simulink model "test_com_SensorFusion_SF_D4_slip_GPS_ukf"  (R2019b)
settings: Solver=FixedStepDiscrete  StartTime=0  StopTime=stop  FixedStep=0.001  RelTol=1e-3
undefined symbols (not defined in the file or in its folder): BxTM, ByTM, CxTM, CyTM, g, gamma_stat_front, gamma_stat_rear, gearbox_ratio, l_F, l_R, m_sprung, m_unsprung_quarter, mag_calib_front_center, mag_calib_front_compmatrix, mag_calib_rear_center, mag_calib_rear_compmatrix, should_be_in_theSensorFusion, switch_VelYcalculation_pSF, testStart_VelX_pSF, testVelY_pSF, tire_r_dyn, track_angle_front, track_width_front, track_width_rear, v2o_x, wheel_kinematics_breakpoints, wheel_kinematics_FL_data, wheel_kinematics_FR_data, wheelbase, x9DFrontX, x9DFrontY, x9DRearX, x9DRearY
libraries: SignalProcessingSensorFusionLib x30, simulink x6
(part 6 of 8)

== matlab function test_com_SensorFusion_SF_D4_slip_GPS_ukf/Subsystem14/SensorFusion_E10/kalman ==
  data: YawRateCalculated output; x9DFront input; x9DRear input; VehicleState output Bus: control_VehicleState size=1; state output single size=22; Covariance output single; v2o input; WheelSpeeds input; WheelSpeeds_Sq input; RockerAngle input; RockerAngle_Sq input; dt input; x9DFrontX parameter; x9DRearX parameter; v2o_x parameter; track_width_front parameter; track_width_rear parameter; z_output output single; TireLoad output; m_sprung parameter; m_unsprung_quarter parameter; l_R parameter; l_F parameter; wheelbase parameter; h_cg parameter; motion_ratio_front parameter; motion_ratio_rear parameter; motion_ratio_heave_front parameter; motion_ratio_heave_rear parameter; motion_ratio_roll_front parameter; motion_ratio_roll_rear parameter; spring_stiff_heave_front parameter; spring_stiff_heave_rear parameter; spring_stiff_roll_front parameter; spring_stiff_roll_rear parameter; damp_coef_heave_front_push parameter size=[1 3]; damp_coef_heave_front_pull parameter size=[1 3]; damp_coef_heave_rear_push parameter size=[1 3]; damp_coef_heave_rear_pull parameter size=[1 3]; damp_coef_roll_front_push parameter size=[1 3]; damp_coef_roll_front_pull parameter size=[1 3]; damp_coef_roll_rear_push parameter size=[1 3]; damp_coef_roll_rear_pull parameter size=[1 3]; g parameter; tire_r_dyn parameter; delta input; Output output; TireSlipLong output; TireSlipAngle output; bias output; measurements_nb_out output; Position_out output; WheelAngle_FL input; WheelAngle_FR input; RockerAngle_nb output; WheelVelocity output; Fx_wheel_wheel input single size=4; Fy_wheel_wheel input single size=4; c_Reib input; rho_air parameter; cdA parameter; clA_front parameter; clA_rear parameter; x9D_Front_AccX_nb output; x9D_Rear_AccX_nb output; kalman_is_running output; switch_VelYcalculation_pSF input; testVelY_pSF input; testStart_VelX_pSF input
function [YawRateCalculated, VehicleState, state, Covariance, z_output , TireLoad, Output, TireSlipLong, TireSlipAngle,...
    bias,measurements_nb_out,Position_out, ...
    RockerAngle_nb, WheelVelocity, x9D_Front_AccX_nb, x9D_Rear_AccX_nb, kalman_is_running]    ...										
    = kalman(x9DFront, x9DRear, v2o, WheelSpeeds, WheelSpeeds_Sq, RockerAngle, RockerAngle_Sq,...
    dt, x9DFrontX, x9DRearX, v2o_x, track_width_front, track_width_rear, ...
    m_sprung,  m_unsprung_quarter, l_R, l_F, wheelbase, h_cg, motion_ratio_front, motion_ratio_rear, ...
    motion_ratio_heave_front, motion_ratio_heave_rear, motion_ratio_roll_front, motion_ratio_roll_rear, ...
    spring_stiff_heave_front, spring_stiff_heave_rear, spring_stiff_roll_front, spring_stiff_roll_rear, ...
    damp_coef_heave_front_push, damp_coef_heave_front_pull, damp_coef_heave_rear_push, damp_coef_heave_rear_pull,...
    damp_coef_roll_front_push, damp_coef_roll_front_pull, damp_coef_roll_rear_push, damp_coef_roll_rear_pull, ...
    g, tire_r_dyn, delta, WheelAngle_FL, WheelAngle_FR, Fx_wheel_wheel, Fy_wheel_wheel,...
    c_Reib, rho_air, cdA, clA_front, clA_rear, switch_VelYcalculation_pSF, testVelY_pSF, testStart_VelX_pSF)


persistent x P
%persistent x_TireLoad P_TireLoad
									
persistent WheelSpeedsCloseTogether_counter WheelSpeedsNoJump_counter
persistent WheelVelocity_old yawRate_old rollAng_old pitchAng_old PosZ_old v2o_VelX_old
persistent TireLoad_old

%Variablen für bias Messung
persistent standstill_counter
persistent bias_measurements 
persistent P_bias



%% Setup

% kalman filter
% x_k+1 = F x_k + w_k
% z_k = H x_k + v_k

% State vector 

% x = [ PosX;           % (1)   x-coordinate of the car  
%       VelX;           % (2)   Velocity of the car in x-direction 
%       AccX;           % (3)   Acceleration in x-direction of the car (CG) 
%       PosY;           % (4)   y-coordinate of the car 
%       VelY;           % (5)   Velocity of the car in y-direction 
%       AccY;           % (6)   Acceleration in y-direction of the car (CG) 
%       PosZ;           % (7)   z-coordinate of the car 
%       VelZ;           % (8)   Velocity of the car in z-direction 
%       AccZ;           % (9)   Acceleration in z-direction of the car (CG) 
%       RollAng;        % (10)  RollAngle of the Monocoque 
%       RollRate;       % (11)  RollRate of the Monocoque 
%       RollAcc;        % (12)  RollAcceleration of the Monocoque 
%       PitchAng;       % (13)  PitchAngle of the Monocoque 
%       PitchRate;      % (14)  PitchRate of the Monocoque 
%       PitchAcc;       % (15)  PitchAcceleration of the Monocoque  
%       YawAng;         % (16)  YawAngle of the Monocoque 
%       YawRate;        % (17)  YawRate of the Monocoque 
%       YawAcc;         % (18)  YawAcceleration of the Monocoque  
%       WheelVelocity_FL;   % (19)  wheelvelocity in m/sec in Rad_KS     
%       WheelVelocity_FR;   % (20)  wheelspeed front right wheel in rad 
%       WheelVelocity_RL;   % (21)  wheelspeed rear  left  wheel in rad 
%       WheelVelocity_RR;   % (22)  wheelspeed rear  right wheel in rad



%%
num_states=22;
num_measurements=23;
YawRate_factor=1; %1.167 Is used since the E9 9D sensors put out yawRate values that were wrong by a factor
if isempty(P)
   
    
    
    %% bias Variablen Initialisierung
    P_bias=eye(num_measurements)*0.001;
    standstill_counter=0;
    bias_measurements=single(zeros(num_measurements,1));
    

    

    WheelSpeedsCloseTogether_counter=0;
    WheelSpeedsNoJump_counter=0;
    
    x = single(zeros(num_states,1));
    P = single(zeros(num_states, num_states));
    
	
    yawRate_old=single(0); % this value is for the derivation of the yaw rate 
    WheelVelocity_old=single([0;0;0;0]);
    rollAng_old=single([0;0]);
    pitchAng_old=single([0;0]);
    PosZ_old=single([0;0]);
    v2o_VelX_old=single(0);
    TireLoad_old= single([m_unsprung_quarter+0.5*m_sprung*l_R/wheelbase; ...
        m_unsprung_quarter + 0.5*m_sprung*l_R/wheelbase; ...
        m_unsprung_quarter + 0.5*m_sprung*l_F/wheelbase; ...
        m_unsprung_quarter + 0.5*m_sprung*l_F/wheelbase]);
  
end


%% Readability

    PosX=x(1);
    VelX=x(2);
    AccX=x(3);
    PosY=x(4);
    VelY=x(5);
    AccY=x(6);
    PosZ=x(7);
    VelZ=x(8);
    AccZ=x(9);
    RollAngle=x(10);
    RollRate=x(11);
    RollAcc=x(12);
    PitchAngle=x(13);
    PitchRate=x(14);
    PitchAcc=x(15);
    YawAngle=x(16);
    YawRate=x(17);
    YawAcc=x(18);
    WheelVelocity_FL=x(19);
    WheelVelocity_FR=x(20);
    WheelVelocity_RL=x(21);
    WheelVelocity_RR=x(22);

    

    measurements= [
v2o.VelX            % (1)   v2o Sensor x velocity
v2o.VelY            % (2)   v2o Sensor y velocity
v2o.SlipAngle       % (3)   v2o Sensor Slipangle
x9DFront.AccX       % (4)   IMU Front  x acceleration
x9DFront.AccY       % (5)   IMU Front  y acceleration
x9DFront.AccZ       % (6)   IMU Front  z acceleration
x9DFront.RollRate   % (7)   IMU Front  RollRate
x9DFront.PitchRate  % (8)   IMU Front  PitchRate
x9DFront.YawRate    % (9)   IMU Front  YawRate
x9DRear.AccX        % (10)  IMU Rear   x acceleration
x9DRear.AccY        % (11)  IMU Rear   y acceleration
x9DRear.AccZ        % (12)  IMU Rear   z acceleration
x9DRear.RollRate    % (13)  IMU Rear   RollRate
x9DRear.PitchRate   % (14)  IMU Rear   PitchRate
x9DRear.YawRate     % (15)  IMU Rear   YawRate
WheelSpeeds(1)      % (16)  wheelspeed  FL
WheelSpeeds(2)      % (17)  wheelspeed  FR
WheelSpeeds(3)      % (18)  wheelspeed  RL
WheelSpeeds(4)      % (19)  wheelspeed  RR
RockerAngle(1)      % (20)  Rockerangle FL
RockerAngle(2)      % (21)  Rockerangle FR
RockerAngle(3)      % (22)  Rockerangle RL
RockerAngle(4)      % (23)  Rockerangle RR
];

measurements_Sq= [
v2o.VelX_Sq            % (1)   v2o Sensor x velocity        Signal Quality
v2o.VelY_Sq            % (2)   v2o Sensor y velocity        Signal Quality
v2o.SlipAngle_Sq       % (3)   v2o Sensor Slipangle         Signal Quality
x9DFront.AccX_Sq       % (4)   IMU Front  x acceleration    Signal Quality
x9DFront.AccY_Sq       % (5)   IMU Front  y acceleration    Signal Quality
x9DFront.AccZ_Sq       % (6)   IMU Front  z acceleration    Signal Quality
x9DFront.RollRate_Sq   % (7)   IMU Front  RollRate          Signal Quality
x9DFront.PitchRate_Sq  % (8)   IMU Front  PitchRate         Signal Quality
x9DFront.YawRate_Sq    % (9)   IMU Front  YawRate           Signal Quality
x9DRear.AccX_Sq        % (10)  IMU Rear   x acceleration    Signal Quality
x9DRear.AccY_Sq        % (11)  IMU Rear   y acceleration    Signal Quality
x9DRear.AccZ_Sq        % (12)  IMU Rear   z acceleration    Signal Quality
x9DRear.RollRate_Sq    % (13)  IMU Rear   RollRate          Signal Quality
x9DRear.PitchRate_Sq   % (14)  IMU Rear   PitchRate         Signal Quality
x9DRear.YawRate_Sq     % (15)  IMU Rear   YawRate           Signal Quality
WheelSpeeds_Sq(1)      % (16)  wheelspeed  FL               Signal Quality
WheelSpeeds_Sq(2)      % (17)  wheelspeed  FR               Signal Quality
WheelSpeeds_Sq(3)      % (18)  wheelspeed  RL               Signal Quality
WheelSpeeds_Sq(4)      % (19)  wheelspeed  RR               Signal Quality
RockerAngle_Sq(1)      % (20)  Rockerangle FL               Signal Quality
RockerAngle_Sq(2)      % (21)  Rockerangle FR               Signal Quality
RockerAngle_Sq(3)      % (22)  Rockerangle RL               Signal Quality
RockerAngle_Sq(4)      % (23)  Rockerangle RR               Signal Quality
];


%Correction of the sensor inputs with the estimated biases
% nb == no bias
measurements_nb=    measurements-bias_measurements;
WheelSpeeds_nb=     single(zeros(4,1));
RockerAngle_nb=     single(zeros(4,1));
    
v2o_VelX_nb=            measurements_nb(1);
v2o_VelY_nb=            measurements_nb(2);
v2o_SlipAngle_nb=       measurements_nb(3);
x9D_Front_AccX_nb=      measurements_nb(4);
x9D_Front_AccY_nb=      measurements_nb(5);
x9D_Front_AccZ_nb=      measurements_nb(6);     %Gravitation berücksichtigen ???
x9D_Front_RollRate_nb=  measurements_nb(7);
x9D_Front_PitchRate_nb= measurements_nb(8);
x9D_Front_YawRate_nb=   measurements_nb(9)*YawRate_factor;
x9D_Rear_AccX_nb=       measurements_nb(10);
x9D_Rear_AccY_nb=       measurements_nb(11);
x9D_Rear_AccZ_nb=       measurements_nb(12);    %Gravitation berücksichtigen ???
x9D_Rear_RollRate_nb=   measurements_nb(13);
x9D_Rear_PitchRate_nb=  measurements_nb(14);
x9D_Rear_YawRate_nb=    measurements_nb(15)*YawRate_factor;
WheelSpeeds_nb(1)=      measurements_nb(16);
WheelSpeeds_nb(2)=      measurements_nb(17);
WheelSpeeds_nb(3)=      measurements_nb(18);
WheelSpeeds_nb(4)=      measurements_nb(19);
RockerAngle_nb(1)=      measurements_nb(20);
RockerAngle_nb(2)=      measurements_nb(21);
RockerAngle_nb(3)=      measurements_nb(22);
RockerAngle_nb(4)=      measurements_nb(23);

Fx_wheel_vehicle=single([1; 1; 1; 1]);
Fy_wheel_vehicle=single([1; 1; 1; 1]);

Fx_wheel_vehicle(1)=cos(WheelAngle_FL)*Fx_wheel_wheel(1)-sin(WheelAngle_FL)*Fy_wheel_wheel(1);
Fx_wheel_vehicle(2)=cos(WheelAngle_FR)*Fx_wheel_wheel(2)-sin(WheelAngle_FR)*Fy_wheel_wheel(2);
Fy_wheel_vehicle(1)=sin(WheelAngle_FL)*Fx_wheel_wheel(1)+cos(WheelAngle_FL)*Fy_wheel_wheel(1);
Fy_wheel_vehicle(2)=sin(WheelAngle_FR)*Fx_wheel_wheel(2)+cos(WheelAngle_FR)*Fy_wheel_wheel(2);
Fx_wheel_vehicle(3:4)=Fx_wheel_wheel(3:4);
Fy_wheel_vehicle(3:4)=Fy_wheel_wheel(3:4);

F_aeroFz     = 0.5  * rho_air * clA_front * (VelX^2+AccX^2) ;
F_aeroRz     = 0.5  * rho_air * clA_rear * (VelX^2+AccX^2)  ;
F_aerox      = 0.5  * rho_air * cdA   * (VelX^2+AccX^2)  ;    
F_wheel_reib = -c_Reib*TireLoad_old.*(TireLoad_old>0);
sum_F_wheel_reib=F_wheel_reib(1)+F_wheel_reib(2)+F_wheel_reib(3)+F_wheel_reib(4);								  
									  																			 %% Preparing WheelSpeeds

% Differenz durchschnittl. Raddrehzahl / Schwimmwinkelsensor > Schwellwert
% -> Schwimmwinkelsensor nicht vertrauen

WheelVelocity = WheelSpeeds * tire_r_dyn; % dynamischer Reifenradius

% Durchschnittliche Radgeschwindigkeiten ermitteln
avgWheelVelocity = mean(WheelVelocity);
%(WheelSpeeds.WheelSpeed_FL + WheelSpeeds.WheelSpeed_FR + WheelSpeeds.WheelSpeed_RL + WheelSpeeds.WheelSpeed_RR) / 4;
avarageWheelVelocity=single(avgWheelVelocity);


WheelDistances = [-track_width_front/2; track_width_front/2; ...
    -track_width_rear/2; track_width_rear/2];
WheelVelocity_CoG=WheelVelocity+WheelDistances*x(17);  %x17 YawRate
WheelVelocity_CoG(1)=WheelVelocity_CoG(1)*cos(WheelAngle_FL);
WheelVelocity_CoG(2)=WheelVelocity_CoG(2)*cos(WheelAngle_FR);

MinWheelVelocity = min(WheelVelocity_CoG);
MaxWheelVelocity = max(WheelVelocity_CoG);


if((max(abs(WheelVelocity-WheelVelocity_old))/dt)<10)
    WheelSpeedsNoJump_counter=WheelSpeedsNoJump_counter+1;
else
    WheelSpeedsNoJump_counter=0;
end
if(MaxWheelVelocity-avgWheelVelocity<0.6 && avgWheelVelocity-MinWheelVelocity<0.6)
    WheelSpeedsCloseTogether_counter=WheelSpeedsCloseTogether_counter+1;
else
    WheelSpeedsCloseTogether_counter=0;
end


%% valueIsNew Slipangle Sensor
valueIsNew = false;
if(v2o_VelX_old~=v2o_VelX_nb)
    valueIsNew = true;
    v2o_VelX_old=v2o_VelX_nb;
end


%% Prediction 

if(avgWheelVelocity < 0.01 )
        vehicle_is_driving=false;
        standstill_counter=standstill_counter+1;
    else
        vehicle_is_driving=true;
        standstill_counter=0;
end
bias_measurement=false;
kalman_is_running=false;
if ~vehicle_is_driving
    
    if standstill_counter*dt>0.5 && standstill_counter*dt<10
    bias_measurement=true;    
    kill_matrix_bias=zeros(num_measurements,num_measurements);
        for i=1:num_measurements
            if measurements_Sq(i)<4
                kill_matrix_bias(i,i)=1;
            end
        end
%         kill_matrix_bias=zeros(num_measurements,num_measurements);
        H_bias=kill_matrix_bias;
        R_bias=eye(num_measurements)*0.01;  % Sinnvolle Werte?
        I_bias=eye(num_measurements);
        
        Z_bias = kill_matrix_bias*measurements;
        w_bias = Z_bias-(H_bias*bias_measurements);
        K_bias = (P_bias*H_bias')/(H_bias*P_bias*H_bias.'+R_bias);  
        bias_measurements = bias_measurements+K_bias*w_bias;
        P_bias = (I_bias-K_bias*H_bias)*P_bias;
    end

    else % update the state only if the biases are currently not measured
    kalman_is_running=true;
    sum_Fx=Fx_wheel_vehicle(1)+Fx_wheel_vehicle(2)+Fx_wheel_vehicle(3)+Fx_wheel_vehicle(4);
    sum_Fy=Fy_wheel_vehicle(1)+Fy_wheel_vehicle(2)+Fy_wheel_vehicle(3)+Fy_wheel_vehicle(4);
    % nonlinear system-equotations
   x=[ PosX+cos(YawAngle)*dt*VelX-sin(YawAngle)*VelY*dt;    % (1)    PositionX       
		%VelX+dt*((sum_Fx+sum_F_wheel_reib-F_aerox)/(m_sprung+m_unsprung_quarter*4)); %+VelY*YawRate																						 
        VelX+dt*(AccX+VelY*YawRate);                          % (2)   Velocity in x-direction          
        AccX;                                               %  AccX(3)   Acceleration in x-direction of the car (CG)
        PosY+VelX*dt*sin(YawAngle)+dt*VelY*cos(YawAngle);   % (4) Position in y_Richtung								
									
        VelY+dt*(AccY-VelX*YawRate);                          % VelY(5)   Velocity in y-direction 	   
			   
        AccY;                                               %  AccY; % (6)   Acceleration in y-direction       
        PosZ;                                       % PosZ; (7)   position of the car in z-direction                
        VelZ;                                               % VelZ;(8)   velocity of the car in z-direction               
        AccZ;                                               % AccZ;(9)   Acceleration in z-direction of the car (CG)             
        RollAngle+0*RollRate;                                              % RollAng; (10)   RollAngle of the Monocoque             
        RollRate+0*RollAcc;                                     % RollRate; (11)   RollRate of the Monocoque            
        RollAcc;                                              % RollAcc;(12)  RollAcceleration of the Monocoque
        PitchAngle;                                              % PitchAng;(13)  PitchAngle of the Monocoque        
        x(14)+dt*x(15);                                     % PitchRate;(14)  PitchRate of the Monocoque             
        x(15);                                              %  PitchAcc;(15)  PitchAcceleration of the Monocoque 
        x(16)+dt*x(17);                                     % YawAng;  (16)   YawAngle of the Monocoque
        x(17)+dt*x(18);                                              %  YawRate;(17)   YawRate of the Monocoque                
        x(18);                                              % YawAcc;(18)  YawAcceleration of the Monocoque          
        x(19);                                              % wheelVelocity_FL;(19)  wheelspeed front left  wheel in rad         
        x(20);                                              %  wheelVelocity_FR;(20)  wheelspeed front right wheel in rad         
        x(21);                                              % wheelVelocity_RL;(21)  wheelspeed rear  left  wheel in rad           
        x(22)];                                              % wheelVelocity_RR;(22)  wheelspeed rear  right wheel in rad ];                                             %Vely classic                       


    %Calculating a linearized A Matrix
          %PosX           VelX                AccX          PosY
          %VelY        AccY PosZ        VelZ          AccZ RollAngle
          %RollRate  RollAcc PitchAn PitchRate PitchAcc  YawAngle                                    YawRate YawAcc  19  20  21  22 
    A=[ 1,  cos(YawAngle)*dt,                0,             0,   -sin(YawAngle)*dt,  0,  0,           0,             0,  0,           0,          0,  0,  0,           0,  -sin(YawAngle)*dt*VelX-cos(YawAngle)*dt*VelY,    0,       0,  0,  0,  0,  0; %PosX  
        0,               1,                  dt,            0,         dt*YawRate,   0,  0,           0,             0,  0,           0,          0,  0,  0,           0,          0,                                      dt*VelY,  0,  0,  0,  0,  0; %VelX 
        0,               0,                  1,             0,         0,            0,  0,           0,             0,  0,           0,          0,  0,  0,           0,          0,                                       0,       0,  0,  0,  0,  0; %AccX 
        0 dt*sin(YawAngle),                  0,             1,    dt*cos(YawAngle),  0,  0,           0,             0,  0,           0,          0,  0,  0,            0,  cos(YawAngle)*dt*VelX-dt*sin(YawAngle)*VelY,    0,       0,  0,  0,  0,  0; %PosY
        0,     -dt*YawRate,                  0,             0,         1,            dt, 0,           0,             0,  0,           0,          0,  0,  0,           0,         0,                                   -dt*VelX,    0,  0,  0,  0,  0; %VelY
        0,               0,                  0,             0,         0,            1,  0,           0,             0,  0,           0,          0,  0,  0,           0,          0,                                       0,       0,  0,  0,  0,  0; %AccY
        0,               0,                  0,             0,         0,            0,  1,           0,             0,  0,           0,          0,  0,  0,           0,           0,                                       0,       0,  0,  0,  0,  0; %PosZ
        0,               0,                  0,             0,         0,            0,  0,           1,             0,  0,           0,          0,  0,  0,           0,          0,                                       0,       0,  0,  0,  0,  0; %VelZ
        0,               0,                  0,             0,         0,            0,  0,           0,             1,  0,           0,          0,  0,  0,           0,          0,                                       0,       0,  0,  0,  0,  0; %AccZ
        0,               0,                  0,             0,         0,            0,  0,           0,             0,  1,          0,          0,  0,  0,           0,          0,                                       0,       0,  0,  0,  0,  0; %RollAngle
        0,               0,                  0,             0,         0,            0,  0,           0,             0,  0,           1,          0,  0,  0,          0,          0,                                       0,       0,  0,  0,  0,  0; %RollRate
        0,               0,                  0,             0,         0,            0,  0,           0,             0,  0,           0,          1,  0,  0,           0,          0,                                       0,       0,  0,  0,  0,  0; %RollAcc
        0,               0,                  0,             0,         0,            0,  0,           0,             0,  0,           0,          0,  1,  0,           0,          0,                                       0,       0,  0,  0,  0,  0; %PitchAngle 
        0,               0,                  0,             0,         0,            0,  0,           0,             0,  0,           0,          0,  0,  1,           dt,          0,                                       0,       0,  0,  0,  0,  0; %PitchRate
        0,               0,                  0,             0,         0,            0,  0,           0,             0,  0,           0,          0,  0,  0,           1,          0,                                       0,       0,  0,  0,  0,  0; %PitchAcc
        0,               0,                  0,             0,         0,            0,  0,           0,             0,  0,           0,          0,  0,  0,           0,          1,                                       dt,       0,  0,  0,  0,  0; %YawAngle
        0,               0,                  0,             0,         0,            0,  0,           0,             0,  0,           0,          0,  0,  0,           0,          0,                                       1,       dt,  0,  0,  0,  0; %YawRate
        0,               0,                  0,             0,         0,            0,  0,           0,             0,  0,           0,          0,  0,  0,           0,          0,                                       0,       1,  0,  0,  0,  0; %YawAcc
        0,               0,                  0,             0,         0,            0,  0,           0,             0,  0,           0,          0,  0,  0,           0,          0,                                       0,       0,  1,  0,  0,  0; %WheelspeedFL
        0,               0,                  0,             0,         0,            0,  0,           0,             0,  0,           0,          0,  0,  0,           0,          0,                                       0,       0,  0,  1,  0,  0; %WheelspeedFR
        0,               0,                  0,             0,         0,            0,  0,           0,             0,  0,           0,          0,  0,  0,           0,          0,                                       0,       0,  0,  0,  1,  0; %WheelspeedRL
        0,               0,                  0,             0,         0,            0,  0,           0,             0,  0,           0,          0,  0,  0,           0,          0,                                       0,       0,  0,  0,  0,  1];%WheelspeedRR
        %VelY]; 



    W = eye(num_states);

%     exp=single(0.4/((0.2*(x(5)-1)^2)+1)-2.4);%(0.4*(2^(-0.1*(x(5)-1)^2))-3.1);%-2.7*2^(-0.1*(x(5)-1)^2)-3.1*(-2^(-0.1*(x(5)-1)^2)+1) % This exponent is a value between -2.1 (if x(5)=2) and -4.5 (if x(5) is away from 2)
    % Covariance matrix of state noise
 Q = diag([0.0001;        %Positionx (1)
            0.001;        %VelX;   (2)   Velocity in x
            0.001;        %AccX;   (3)   Acceleration in x-direction of the car (CG)4
            0.01;         %PositionY  (4)
            0.001;             %Velocity in y;      (5)  
            0.0001;        %AccY;               (6) in y-direction  
            0.0001;        %PosZ;               (7)   position of the car in z-direction
            0.00005;        %VelZ;               (8)   velocity of the car in y-direction
            0.00001;       %AccZ;               (9)   Acceleration in x-direction of the car (CG)
            0.00001;       %RollAng;         % (10)   RollAngle of the Monocoque
            0.00001;        %RollRate;        % (11)   RollRate of the Monocoque
            0.0002;        %RollAcc;         % (12)  RollAcceleration of the Monocoque 
            0.00001;       %PitchAng;        % (13)  PitchAngle of the Monocoque
            0.0001;        %PitchRate;       % (14)  PitchRate of the Monocoque
            0.0002;        %PitchAcc;        % (15)  PitchAcceleration of the Monocoque 
            0.01;          %YawAng;          % (16)   YawAngle of the Monocoque
            0.001;       %YawRate;         % (17)   YawRate of the Monocoque
            0.001;         %YawAcc;          % (18)  YawAcceleration of the Monocoque 
            0.008;       %WheelspeedFL;    % (19)  
            0.008;       %WheelspeedFR;    % (20)  
            0.008;       %WheedspeedRL;    % (21)  
            0.008]*0.002);           %WheelspeedRR;    % (22)   %dt
             
            

    % prediction calculation
    %x = x + dt*F*x; % + dt*B*u;          % statevector update
    %NO LINEAR EQUOTATION USED, THEREFORE ONLY THE LINEARIZED MATRIX A IS USED
    %TO UPDATE P

    P = A*P*A' + W*Q*W';                 % covariance matrix update
				   
end 

%% calculating turning Radius of car for Pfuschlösung if all 9D  or slipanglesensor
   if (abs((WheelAngle_FL+WheelAngle_FR)*0.5)>pi/180)
     r_y=single((wheelbase-VelX*0.03+0.0)*tan(sign((WheelAngle_FL+WheelAngle_FR)*0.5)*(pi*0.5)-0.2047*3.76*((WheelAngle_FL+WheelAngle_FR)*0.5))); %TODO nachvollziehen, Radius über delta und VelX
   else
     r_y=single(9999999);
   end
   
if(avgWheelVelocity < 0.01 )
    VelX=single(0);
    VelY=single(0);
end

H_oben= eye(22);

h1=[ x; 
    PosZ-l_F*PitchAngle-RollAngle*0.5*track_width_front; 
    PosZ-l_F*PitchAngle+RollAngle*0.5*track_width_front;
    PosZ+l_R*PitchAngle-RollAngle*0.5*track_width_rear;
    PosZ+l_R*PitchAngle+RollAngle*0.5*track_width_rear];
%% Measurement SF
% Measurement selection: With the help of the singal qualifiers it is
% determined which signal can be used as a measurement input for the kalman
% filter
%% Start der States
% Position X wird später bei uns von GPS gemessen noch kein info wie genau,
% bei Start wird Position auf null gesetzt

if(avgWheelVelocity < 0.01 )
    VelX=single(0);
    VelY=single(0);
end 
if( avgWheelVelocity< 1.5) && testStart_VelX_pSF==true
    VelX=v2o_VelX_nb;
end 


PosX_CoG_measurement=PosX;
R_PosX=0.01;
selection=[];
%% Wertberechnung (2) von Velx mit Ersatzlösungen je nach Signal Qualifier
	Option_VelX=0;		  
if (v2o.VelX_Sq<4) && (v2o.VelY_Sq<4) && abs(v2o_VelX_nb-v2o_VelX_old) < 2
    VelX_CoG_measurement=v2o_VelX_nb; %-YawRate*v2o_x;  wie bei E9 vernachlässigbar
    R_VelX=0.00001;
        if VelX<2.5 && VelX>1.3
       zeta=(VelX-1.1)/(2.5-1.3); 
        R_VelX=0.01*zeta+(1-zeta)*0.00001;
    elseif VelX<1.3
        R_VelX=single(0.01);
    else
       R_VelX=single(0.00001);
    end
    selection=[selection 2];
	Option_VelX=1;	  
elseif ((v2o.VelX_Sq>3) || abs(v2o_VelX_nb-v2o_VelX_old) > 2) && (MaxWheelVelocity-avgWheelVelocity<5 && avgWheelVelocity-MinWheelVelocity<5)
    if AccX>0 % Beschleunigen 
    VelX_CoG_measurement=MinWheelVelocity;
    R_VelX=single(0.001);
    selection=[selection 2];
	Option_VelX=2;			  
    else 
    VelX_CoG_measurement= single(MaxWheelVelocity);
    R_VelX=single(0.001);
    selection=[selection 2];
	Option_VelX=3;			  
    end
else
    VelX_CoG_measurement=single(0); %wird nicht verwendet
    R_VelX=single(0.01);
end



%% für AccX (3) gemessene Werte 
if (x9DFront.AccX_Sq<4)&&(x9DRear.AccX_Sq<4)
 AccX_CoG_measurement=((x9D_Front_AccX_nb+x9D_Rear_AccX_nb)/2.0)+AccZ*PitchAngle; %linearisierte Gleichung gerollt in ungerollt, von Vehicle zu Orientierung Inertialsystem
    R_AccX=0.00001;
    selection=[selection 3];
elseif (x9DFront.AccX_Sq<4)&&(x9DRear.AccX_Sq>3)
    AccX_CoG_measurement=(x9D_Front_AccX_nb)+AccZ*PitchAngle;%+x9DFrontX*YawRate^2;%accZ noch und pitch
    R_AccX=0.00001;
    selection=[selection 3];
elseif (x9DFront.AccX_Sq>3)&&(x9DRear.AccX_Sq<4)
    AccX_CoG_measurement=(x9D_Rear_AccX_nb)+AccZ*PitchAngle;
    R_AccX=0.00001;
    selection=[selection 3];
elseif (x9DFront.AccX_Sq>3)&&(x9DRear.AccX_Sq>3)&& (MaxWheelVelocity-avgWheelVelocity<0.6 && avgWheelVelocity-MinWheelVelocity<0.6)
   AccX_CoG_measurement=(avgWheelVelocity-mean(WheelVelocity_old))/dt;
   R_AccX=0.1;
   selection=[selection 3];
else 
    AccX_CoG_measurement=single(0);
    R_AccX=0.01;
end


%hier aktuell keine MEsswerte
PosY_CoG_measurement=PosY;
R_PosY=0.1;



% VelY (5)
if testVelY_pSF==0
 v2o.VelY_Sq=uint8(22);
else
    v2o.VelY_Sq=v2o.VelY_Sq;
end   
VelY_CoG_measurement=single(0);
sum_Fy=Fy_wheel_vehicle(1)+Fy_wheel_vehicle(2)+Fy_wheel_vehicle(3)+Fy_wheel_vehicle(4);																					   

%VelY klassic kalman filter
if (v2o.VelY_Sq<4) && switch_VelYcalculation_pSF==0
    VelY_CoG_measurement=v2o_VelY_nb-YawRate*v2o_x; % Vely minus YawRate*Hebelarm
    R_VelY=0.00001;
    selection=[selection 5];
elseif  (v2o.VelY_Sq<4)&& switch_VelYcalculation_pSF==1
    VelY_CoG_measurement=v2o_VelY_nb; % Vely minus YawRate*Hebelarm
    R_VelY=0.00001;
    selection=[selection 5];
    H_oben(5,17)=v2o_x;
    h1(5)=VelY+v2o_x*YawRate;
else  
    VelY_CoG_measurement= 1.6*(dt*((sum_Fy)/(m_sprung+m_unsprung_quarter*4))-v2o_x*YawRate);  %Pfuschlösung mit x(2=VelX
    R_VelY=0.0005; % 0.03 Eigenlenkgradient?
    selection=[selection 5];							 
end


% AccY (6) Berechnung und Signal auswahl
if (x9DFront.AccY_Sq<4)&&(x9DRear.AccY_Sq<4) 
    AccY_CoG_measurement=((x9D_Front_AccY_nb)*abs(x9DRearX)+(x9D_Rear_AccY_nb)*abs(x9DFrontX))/(abs(x9DFrontX)...
        +abs(x9DRearX))-AccZ*RollAngle; 
    R_AccY=0.001;
    selection=[selection 6];
elseif (x9DFront.AccY_Sq<4)&&(x9DRear.AccY_Sq>3)
    AccY_CoG_measurement= ((x9D_Front_AccY_nb)+YawRate^2*(x9DFrontX))-AccZ*RollAngle; 
    R_AccY=0.001;
    selection=[selection 6];
elseif (x9DFront.AccY_Sq>3)&&(x9DRear.AccY_Sq<4)    
    AccY_CoG_measurement= ((x9D_Rear_AccY_nb)+YawRate^2*(x9DRearX))-AccZ*RollAngle;   
    R_AccY=0.001;
    selection=[selection 6];
else
    AccY_CoG_measurement=(VelX^2)/r_y; %x(2) VelX
    R_AccY=0.01;
    selection=[selection 6];
end

% Position Z (7)
PosZ_CoG_measurement=single(0);
R_PosZ=0.01;


% VelZ (8)
VelZ_CoG_measurement= (PosZ-PosZ_old(2))/(dt*2);
R_VelZ=0.1;
selection=[selection 8];

%Für AccZ_CoG (9) aus Messwerten
if (x9DFront.AccZ_Sq<4)&&(x9DRear.AccZ_Sq<4)
    AccZ_CoG_measurement=((x9D_Front_AccZ_nb)*abs(x9DRearX)+(x9D_Rear_AccZ_nb)*abs(x9DFrontX))/(abs(x9DFrontX)+abs(x9DRearX));
    R_AccZ=0.001;
    selection=[selection 9];
else 
    AccZ_CoG_measurement=single(0);
    R_AccZ=0.1;
end

% RollAngle (10)
RollAngle_measurement=single(0);
R_RollAngle=0.1; 


if RockerAngle_Sq(1)<4 ||   RockerAngle_Sq(2)<4 || RockerAngle_Sq(3)<4 || RockerAngle_Sq(4)<4&&(x9DFront.RollRate_Sq>-1) && (x9DRear.RollRate_Sq>-1)														  
    RollRate_measurement=(RollAngle-rollAng_old(2))/(2*dt);  
    R_RollRate=0.1;
    selection=[selection 11];
% elseif (RockerAngle_Sq(1)>4 && RockerAngle_Sq(2)>4 && RockerAngle_Sq(3)>4 && RockerAngle_Sq(4)>4) &&(x9DFront.RollRate_Sq<4) && (x9DRear.RollRate_Sq<4)
%     RollRate_Front=x9D_Front_RollRate_nb;  %plus bias immer 
%     RollRate_Rear=x9D_Rear_RollRate_nb;
%     RollRate_measurement=(RollRate_Front+RollRate_Rear)/2;
%     R_RollRate=20;
%     selection=[selection 11];
% elseif RockerAngle_Sq(1)>4 && RockerAngle_Sq(2)>4 && RockerAngle_Sq(3)>4 && RockerAngle_Sq(4)>4 &&(x9DFront.RollRate_Sq>3) && (x9DRear.RollRate_Sq<4)
%     RollRate_Rear=x9D_Rear_RollRate_nb;
%     RollRate_measurement=RollRate_Rear;
%     R_RollRate=0.01;
%     selection=[selection 11];
% elseif RockerAngle_Sq(1)>4 && RockerAngle_Sq(2)>4 && RockerAngle_Sq(3)>4 && RockerAngle_Sq(4)>4 &&(x9DFront.RollRate_Sq<4) && (x9DRear.RollRate_Sq>3)
%     RollRate_Front=x9D_Front_RollRate_nb;
%     RollRate_measurement=RollRate_Front;
%     R_RollRate=0.01;
%     selection=[selection 11];
else
    RollRate_measurement=single(0);
    R_RollRate=0.1;
end

%RollAcceleration (12)
RollAcc_measurement=RollAcc;
R_RollAcc=0.1;

%PitchAngle (13) 
PitchAngle_measurement=single(0);
R_PitchAngle=0.1;

    
% Pitchrate (14)
% if (x9DFront.PitchRate_Sq<4)&& (x9DRear.PitchRate_Sq<4)
%    PitchRate_Front=x9D_Front_PitchRate_nb;
%    PitchRate_Rear=x9D_Rear_PitchRate_nb;
%    R_PitchRate=0.1;
%    PitchRate_measurement=0.5*(PitchRate_Front+PitchRate_Rear);
% elseif (x9DFront.PitchRate_Sq>3)&& (x9DRear.PitchRate_Sq<4)
%     PitchRate_measurement=x9D_Rear_PitchRate_nb;
%     R_PitchRate=0.01;
% elseif (x9DFront.PitchRate_Sq<4)&& (x9DRear.PitchRate_Sq>3)
%     PitchRate_measurement=x9D_Front_PitchRate_nb;
%     R_PitchRate=0.01;
% else 
    PitchRate_measurement=(PitchAngle-pitchAng_old(2))/(2*dt);
    R_PitchRate=0.1;
    selection=[selection 14];
% end

% PitchAcceleration (15), da hier nicht abhängig von Messung keine Auswahl
PitchAcc_measurement=(x9D_Front_AccZ_nb-(x9D_Rear_AccZ_nb))/(abs(x9DFrontX) +abs(x9DRearX));
R_PitchAcc=0.01;
selection=[selection 11];

% YawAngle (16)  
YawAngle_measurement=single(0);
R_YawAngle=1000;

% YawRate (17) beide 9DSensoren

% YawRate_measurement=(AccY/VelX);
% R_YawRate=0.002;
% selection=[selection 17];
% % if (x9DFront.AccY_Sq<4) && (x9DRear.AccY_Sq<4)
% %     YawRate_measurement=AccY/VelX;
% %     R_YawRate=0.002;
%     selection=[selection 17];
% YawRate_losung=1;
% if (v2o.VelX_Sq<4)&&(x9DFront.AccY_Sq<4) && (x9DRear.YawRate_Sq<4)&&(x9DFront.YawRate_Sq>0) && (x9DRear.YawRate_Sq>0)
%     YawRate_measurement=((x9D_Front_AccY_nb)*abs(x9DRearX)+(x9D_Rear_AccY_nb)*abs(x9DFrontX))/(abs(x9DFrontX)...
%         +abs(x9DRearX))/v2o_VelX_nb;
%     R_YawRate=0.002;
%     selection=[selection 17];
%     YawRate_losung=2;
if (x9DFront.YawRate_Sq<4) && (x9DRear.YawRate_Sq<4)
   YawRate_measurement=0.5*(x9D_Front_YawRate_nb+x9D_Rear_YawRate_nb);
    R_YawRate=0.002;
    selection=[selection 17];
elseif (x9DFront.YawRate_Sq<4) && (x9DRear.YawRate_Sq>3)
    YawRate_measurement=x9D_Front_YawRate_nb;
    R_YawRate=0.002;
    selection=[selection 17];
elseif (x9DRear.YawRate_Sq>3) && (x9DRear.YawRate_Sq<4)
    YawRate_measurement=x9D_Rear_YawRate_nb;
    R_YawRate=0.002;
    selection=[selection 17];
else
    YawRate_measurement=single(0);
    R_YawRate=0.1;
end

% YawAccel (18) 
if (x9DFront.AccY_Sq<4)&&(x9DRear.AccY_Sq<4) 
    YawAcc_measurement=(x9D_Front_AccY_nb - x9D_Rear_AccY_nb)/(abs(x9DFrontX) +abs(x9DRearX)) ; 
    R_YawAcc=0.1;
    selection=[selection 18];
else 
    YawAcc_measurement=(YawRate-yawRate_old)/dt;
    R_YawAcc=0.1;
    selection=[selection 18];
end

% WheelSpeeds (19) Front Left
if WheelSpeeds_Sq(1)<3
    WheelVelocity_FL_measurement=tire_r_dyn*WheelSpeeds_nb(1);
    R_WheelVelocity_FL=0.0001;
    selection=[selection 19];
elseif WheelSpeeds_Sq(1)>4 && WheelSpeeds_Sq(2)<3 && WheelSpeeds_Sq(3)<3 && WheelSpeeds_nb(4)<3
    WheelVelocity_FL_measurement= tire_r_dyn*(WheelSpeeds_nb(2)+WheelSpeeds_nb(3)+WheelSpeeds_nb(4))/3;%tire_r_dyn*
    R_WheelVelocity_FL=0.0001;
    selection=[selection 19];
else
    WheelVelocity_FL_measurement=single(0);
    R_WheelVelocity_FL=0.001;
end

% WheelSpeeds (20) Front Left
if WheelSpeeds_Sq(2)<3
    WheelVelocity_FR_measurement=WheelSpeeds_nb(2)*tire_r_dyn;
    R_WheelVelocity_FR=0.0001;
    selection=[selection 20];
elseif WheelSpeeds_Sq(2)>4 && WheelSpeeds_Sq(1)<3 && WheelSpeeds_Sq(3)<3 && WheelSpeeds_nb(4)<3
    WheelVelocity_FR_measurement= tire_r_dyn*(WheelSpeeds_nb(1)+WheelSpeeds_nb(3)+WheelSpeeds_nb(4))/3;
    R_WheelVelocity_FR=0.0001;
    selection=[selection 20];
else
    WheelVelocity_FR_measurement=single(0);
    R_WheelVelocity_FR=0.1;
end

% WheelSpeeds (21) Front Left
if WheelSpeeds_Sq(3)<3
    WheelVelocity_RL_measurement=tire_r_dyn*WheelSpeeds_nb(3);
    R_WheelVelocity_RL=0.0001;
    selection=[selection 21];
elseif WheelSpeeds_Sq(3)>4 && WheelSpeeds_Sq(1)<3 && WheelSpeeds_Sq(2)<3 && WheelSpeeds_nb(4)<3
    WheelVelocity_RL_measurement= tire_r_dyn*(WheelSpeeds_nb(1)+WheelSpeeds_nb(2)+WheelSpeeds_nb(4))/3;
    R_WheelVelocity_RL=0.0001;
    selection=[selection 21];
else
    WheelVelocity_RL_measurement=single(0);
    R_WheelVelocity_RL=0.0001;
end
% WheelSpeeds (22) Front Left
if WheelSpeeds_Sq(4)<3
    WheelVelocity_RR_measurement=tire_r_dyn*WheelSpeeds_nb(4);
    R_WheelVelocity_RR=0.0001;
    selection=[selection 22];
elseif WheelSpeeds_Sq(4)>4 && WheelSpeeds_Sq(1)<3 && WheelSpeeds_Sq(3)<3 && WheelSpeeds_nb(3)<3
    WheelVelocity_RR_measurement= tire_r_dyn*(WheelSpeeds_nb(1)+WheelSpeeds_nb(3)+WheelSpeeds_nb(3))/3;
    R_WheelVelocity_RR=0.0001;
    selection=[selection 22];
else
  WheelVelocity_RR_measurement=single(0);
    R_WheelVelocity_RR=0.0001;
end


kalman_TireLoad=0;
% für Radhub abhängig von HallSensoren
if (RockerAngle_Sq(1)<4)
	selection=[selection 23];
else
   kalman_TireLoad=kalman_TireLoad+1;
end

if (RockerAngle_Sq(2)<4)
	selection=[selection 24];
else
   kalman_TireLoad=kalman_TireLoad+1;
end

if (RockerAngle_Sq(3)<4)
	selection=[selection 25];
else
   kalman_TireLoad=kalman_TireLoad+1;
end

if (RockerAngle_Sq(4)<4)
	selection=[selection 26];
else
   kalman_TireLoad=kalman_TireLoad+1;
end


if ((RockerAngle_Sq(1)>3)&&(RockerAngle_Sq(2)>3)&&(RockerAngle_Sq(4)<4)&&(RockerAngle_Sq(3)<4))||((RockerAngle_Sq(3)>3)&&(RockerAngle_Sq(4)>3)&&(RockerAngle_Sq(1)<4)&&(RockerAngle_Sq(2)<4))
    delta_h=h_cg*AccX*(m_sprung)/(2*(l_F*motion_ratio_heave_front^2*spring_stiff_heave_front+l_R*motion_ratio_heave_rear^2*spring_stiff_heave_rear));
    if((RockerAngle_Sq(1)>3)) %wenn die vorderen beiden FDS sensoren ausgefallen sind
        RH_RL=(RockerAngle_nb(3))*motion_ratio_rear;                                                                      % (25)   pitch-angle (left)
        RH_RR=(RockerAngle_nb(4))*motion_ratio_rear;
        RH_FL=RH_RL-delta_h;
        RH_FR=RH_RR-delta_h;
        selection= [selection 23 24];
    else
        RH_FL=(RockerAngle_nb(1))*motion_ratio_front;                                                                     % (23)   roll-angle (front)
        RH_FR=(RockerAngle_nb(2))*motion_ratio_front;
        RH_RL=RH_FL+delta_h;
        RH_RR=RH_FR+delta_h;  
        selection= [selection 25 26];
    end
       
else
    RH_FL=(RockerAngle_nb(1))*motion_ratio_front;                                                                     % (23)   roll-angle (front)
     RH_FR=(RockerAngle_nb(2))*motion_ratio_front;                                                                     % (24)   roll-angle (rear)
     RH_RL=(RockerAngle_nb(3))*motion_ratio_rear;                                                                      % (25)   pitch-angle (left)
     RH_RR=(RockerAngle_nb(4))*motion_ratio_rear;  
end


% Measured states
    
z1 = [ PosX_CoG_measurement;    % GPS.PosX (1)
      VelX_CoG_measurement;     % VelX (2) im Schwerpunkt aus gemessenen Werten berechnet
      AccX_CoG_measurement;     % AccX (3) im Schwerpunkt aus gemessenen Werten berechnet
      PosY_CoG_measurement;     % GPS.PosY (4)
      VelY_CoG_measurement;     % VelY (5)
      AccY_CoG_measurement;     % AccY (6) im Schwerpunkt aus gemessenen Werten berechnet
      PosZ_CoG_measurement;     % PositionZ (7)
      VelZ_CoG_measurement;     % VelZ (8) Schwerpunkt aus gemessenen Werten
      AccZ_CoG_measurement;     % AccZ_CoG (9)  
      RollAngle_measurement;    % RollAngle (10)
      RollRate_measurement;     % RollRate (11) 
      RollAcc_measurement;      % RollAcceleration (12)
      PitchAngle_measurement;   % PitchAngle (13)
      PitchRate_measurement;    % PitchRate (14)
      PitchAcc_measurement;     % PitchAcceleration (15)
      YawAngle_measurement;     % YawAngle (16)
      YawRate_measurement;      % YawRate  (17)
      YawAcc_measurement;       % YawAcc (18)
      WheelVelocity_FL_measurement;     % WheelspeedFL (19)
      WheelVelocity_FR_measurement;     %WheelspeedFR  (20)
      WheelVelocity_RL_measurement;     %WheelspeedRL  (21)
      WheelVelocity_RR_measurement;   %WheelspeedRR (22)
      RH_FL;
      RH_FR;
      RH_RL;
      RH_RR];    
  

kill_matrix=zeros(length(z1),length(z1));
z=single(zeros(size(z1)));

for w=1:length(selection)
    z(selection(w))=z1(selection(w));    
    kill_matrix(selection(w),selection(w))=1.0;
end

yawRate_old=YawRate; % Save old yawRate to calculate the yawAcc by derivation
rollAng_old(2)=rollAng_old(1);
rollAng_old(1)=RollAngle;
pitchAng_old(2)=pitchAng_old(1);
pitchAng_old(1)=PitchAngle;
PosZ_old(2)=PosZ_old(1);
PosZ_old(1)=PosZ;
WheelVelocity_old=WheelVelocity;



h=kill_matrix*h1;

R = diag([     
    R_PosX;                       % (1)   x-Acc (front)
    R_VelX;                       % (2)   y-Acc (front)
    R_AccX;                       % (3)   x-Acc (rear)
    R_PosY;                       % (4)   y-Acc (rear)
    R_VelY;                       % (5)   x-Acc (average)
    R_AccY;                       % (6)   y-Acc (average)
    R_PosZ;                       % (7)   z-Acc (average)
    R_VelZ;                        % (8)   roll-rate (front)
    R_AccZ;                        % (9)   roll-rate (rear)
    R_RollAngle;                        % (10)   pitch-rate (front)
    R_RollRate;                        % (11)   pitch-rate (rear)
    R_RollAcc;                     % (12)   yaw-rate (front)
    R_PitchAngle;                     % (13)   yaw-rate (rear)
    R_PitchRate;                     % (14)   velocity (from slip angle)
    R_PitchAcc;                     % (15)   slipangle (beta)
    R_YawAngle;                       % (16)   slip-angle zeroing
    R_YawRate;                      % (17)  pitch-acceleration
    R_YawAcc;                      % (18)  yaw-acceleration (derivation of yaw Rate)
    R_WheelVelocity_FL;                       % (19)  yaw-acceleration
    R_WheelVelocity_FR;                    % (20)  average speed of wheel
    R_WheelVelocity_RL;                    % (21)  speed of slowest wheel
    R_WheelVelocity_RR;                % (22)  speed of fastest wheel
    0.001;                             % für die RH vgl mit RollANgle, PitchANgle und PosZ
    0.001;
    0.001;
    0.001]);                    


       %PosX VelX  AccX PosY VelY AccY PosZ VelZ AccZ RollAngle         RollRate RollAcc   PitchAn PitchRate PitchAcc  YawAngle                                    YawRate YawAcc  19  20  21  22
H_unten=[ 0 ,   0 , 0 ,   0 , 0 ,   0 ,   1 , 0, 0, -track_width_front*0.5,   0 ,   0 ,     -l_F,   0 ,         0 , 0 , 0 ,  0 , 0 , 0 , 0 , 0 ;     
          0 ,   0 , 0 ,   0 , 0 ,   0 ,   1 , 0, 0, track_width_front*0.5,   0 ,   0 ,      -l_F,   0 ,         0 , 0 , 0 ,  0 , 0 , 0 , 0 , 0 ;     
          0 ,   0 , 0 ,   0 , 0 ,   0 ,   1 , 0, 0, -track_width_rear*0.5,   0 ,   0 ,      l_R,    0 ,         0 , 0 , 0 ,  0 , 0 , 0 , 0 , 0 ;     
          0 ,   0 , 0 ,   0 , 0 ,   0 ,   1 , 0, 0, track_width_rear*0.5,   0 ,   0 ,       l_R,    0 ,         0 , 0 , 0 ,  0 , 0 , 0 , 0 , 0] ;    
H1=[H_oben; H_unten];
H=kill_matrix*H1;

% Correction equations
I = eye(length(x));
V = eye(length(z));

K_tmp = P*H'/(H*P*H'+V*R*V');

x = x + K_tmp*(z-h);
P = (I - K_tmp*H)*P;


%% Check Vel
if VelX<0
    VelX=single(0);
end

%% Output 
Position_out=[PosX; PosY];
measurements_nb_out=measurements_nb;
bias=bias_measurements;

if switch_VelYcalculation_pSF==2 && (v2o.VelY_Sq<4)
    VelY=v2o_VelY_nb-YawRate*v2o_x;
end
    

if VelX==0
YawRateCalculated=single(0);
else
YawRateCalculated=AccY/VelX;
end



VehicleState.PosX = PosX;
VehicleState.PosY = PosY;
VehicleState.VelX = VelX;
VehicleState.VelY = VelY;
VehicleState.YawAngle = YawAngle;
VehicleState.YawRate = YawRate;
VehicleState.YawAcc = YawAcc;
VehicleState.AccX = AccX;
VehicleState.AccY = AccY;
VehicleState.AccZ = AccZ;
VehicleState.isDriving = true;

z_output = z;

state=x;
			  
Covariance = single(P);


%% Output TireLoad
% Ausgang
%% Preparation TireLoad
Output=[PosZ; VelZ; RollAngle; RollRate; PitchAngle; PitchRate];
% MonoShock Auswahl Druck/Zug-Stufe
if -PitchRate*l_F + PosZ > 0  %Vorne Druck
    damp_coef_heave_front = damp_coef_heave_front_push;
else                    %Vorne Zug
    damp_coef_heave_front = damp_coef_heave_front_pull;
end

if PitchRate*l_R + PosZ > 0  %Hinten Druck
    damp_coef_heave_rear = damp_coef_heave_rear_push;
else                    %Hinten Zug
    damp_coef_heave_rear = damp_coef_heave_rear_pull;
end


% Rolldämpfer Auswahl Druck/Zug-Stufe
if RollRate < 0             % if Bedingung muss überprüft werden!
    damp_coef_roll_front = damp_coef_roll_front_push;
    damp_coef_roll_rear = damp_coef_roll_rear_push;
else
    damp_coef_roll_front = damp_coef_roll_front_pull;
    damp_coef_roll_rear = damp_coef_roll_rear_pull; 
end
damp_F=@(v,damp_coef)(v*0.5*(damp_coef(2)+damp_coef(3))+sign(v)*(0.5*(damp_coef(2)-damp_coef(3))*(damp_coef(1)-abs(v*sign(v)-damp_coef(1)))));

%Nicht-Lineare Ausgangsmatrix
C_tl = [  (2*motion_ratio_heave_front^2*spring_stiff_heave_front*PosZ+ motion_ratio_heave_front*damp_F(2*motion_ratio_heave_front*VelZ,damp_coef_heave_front)  -track_width_front*motion_ratio_roll_front^2*spring_stiff_roll_front*RollAngle+  motion_ratio_roll_front*damp_F(-track_width_front*motion_ratio_roll_front*RollRate,damp_coef_roll_front)  -2*l_F*motion_ratio_heave_front^2*spring_stiff_heave_front*PitchAngle+  motion_ratio_heave_front*damp_F(-2*l_F*motion_ratio_heave_front*PitchRate,damp_coef_heave_front));
          (2*motion_ratio_heave_front^2*spring_stiff_heave_front*PosZ+ motion_ratio_heave_front*damp_F(2*motion_ratio_heave_front*VelZ,damp_coef_heave_front)+  track_width_front*motion_ratio_roll_front^2*spring_stiff_roll_front*RollAngle+   motion_ratio_roll_front*damp_F(track_width_front*motion_ratio_roll_front*RollRate,damp_coef_roll_front)  -2*l_F*motion_ratio_heave_front^2*spring_stiff_heave_front*PitchAngle+  motion_ratio_heave_front*damp_F(-2*l_F*motion_ratio_heave_front*PitchRate,damp_coef_heave_front));
            (2*motion_ratio_heave_rear^2*spring_stiff_heave_rear*PosZ+    motion_ratio_heave_rear*damp_F(2*motion_ratio_heave_rear*VelZ,damp_coef_heave_rear)     -track_width_rear*motion_ratio_roll_rear^2*spring_stiff_roll_rear*RollAngle+      motion_ratio_roll_rear*damp_F(-track_width_rear*motion_ratio_roll_rear*RollRate,damp_coef_roll_rear)+    2*l_R*motion_ratio_heave_rear^2*spring_stiff_heave_rear*PitchAngle+      motion_ratio_heave_rear*damp_F(2*l_R*motion_ratio_heave_rear*PitchRate,damp_coef_heave_rear));
            (2*motion_ratio_heave_rear^2*spring_stiff_heave_rear*PosZ+    motion_ratio_heave_rear*damp_F(2*motion_ratio_heave_rear*VelZ,damp_coef_heave_rear)+     track_width_rear*motion_ratio_roll_rear^2*spring_stiff_roll_rear*RollAngle+       motion_ratio_roll_rear*damp_F(track_width_rear*motion_ratio_roll_rear*RollRate,damp_coef_roll_rear)+    2*l_R*motion_ratio_heave_rear^2*spring_stiff_heave_rear*PitchAngle+      motion_ratio_heave_rear*damp_F(2*l_R*motion_ratio_heave_rear*PitchRate,damp_coef_heave_rear))];

D_tl = [m_unsprung_quarter + 0.5*m_sprung*l_R/wheelbase; 
        m_unsprung_quarter + 0.5*m_sprung*l_R/wheelbase; 
        m_unsprung_quarter + 0.5*m_sprung*l_F/wheelbase; 
        m_unsprung_quarter + 0.5*m_sprung*l_F/wheelbase]*g;

TireLoad = C_tl  + D_tl;

% m_ges=4*m_unsprung_quarter+m_sprung;
% if isempty(P_TireLoad)
%     P_TireLoad=single(zeros(4,4));
%     x_TireLoad=single([590; 590; 610; 610]);
% end
%     
% if vehicle_is_driving
%     
% %% Achtung!! in prediction ist stat plus dynamische tireload
% x_TireLoad = [ ...
%     m_ges*(l_R*g-h_cg*AccX)*(0.5+(h_cg*AccY/(track_width_front*g)))/(l_F+l_R);
%     m_ges*(l_R*g-h_cg*AccX)*(0.5-(h_cg*AccY/(track_width_front*g)))/(l_F+l_R);
%     m_ges*(l_F*g+h_cg*AccX)*(0.5+(h_cg*AccY/(track_width_rear*g)))/(l_F+l_R);
%     m_ges*(l_F*g+h_cg*AccX)*(0.5-(h_cg*AccY/(track_width_rear*g)))/(l_F+l_R)
%     ];
% % x_TireLoad=x_TireLoad;
% A_TireLoad=eye(4);
% W_TireLoad=eye(4);
% Q_TireLoad=diag(([0.01; 
%             0.01; 
%             0.01; 
%             0.01])*dt);
% P_TireLoad = A_TireLoad.*P_TireLoad*A_TireLoad + W_TireLoad.*Q_TireLoad*W_TireLoad;                 % covariance matrix update                 
% end     
% % Correction equations
% I_TireLoad = eye(length(x_TireLoad));
%  
% h_TireLoad=[C_tl(1)+D_tl(1);
%             C_tl(2)+D_tl(2);
%             C_tl(3)+D_tl(3);
%             C_tl(4)+D_tl(4)];        
%         
% V_TireLoad = eye(length(h_TireLoad));
%  
% z_TireLoad=x_TireLoad;
% H_TireLoad=eye(4);
% R_TireLoad=diag([0.001;
%             0.0001;
%             0.0001;
%             0.0001]);
% K_tmp_TireLoad = P_TireLoad*H_TireLoad'/(H_TireLoad*P_TireLoad*H_TireLoad'+V_TireLoad*R_TireLoad*V_TireLoad');
%  
% x_TireLoad = x_TireLoad + K_tmp_TireLoad*(z_TireLoad-h_TireLoad);
% P_TireLoad = (I_TireLoad - K_tmp_TireLoad*H_TireLoad)*P_TireLoad;
%  
% %%achtung nur die dynamischen Radlasten
% if kalman_TireLoad>=50
%     TireLoad=single(x_TireLoad);
% end
% if kalman_TireLoad>=50 && avgWheelVelocity < 0.01
%    TireLoad= single([590; 590; 610; 610]);
% end


% Begrenzung der Radlast
for n=1:1:4
    if TireLoad(n) > 1800
        TireLoad(n) = 1800;
    elseif TireLoad(n) < 0
        TireLoad(n) = 0;
    end
end

TireLoad_old=TireLoad;					  
%%Friction Estimation
vel = ([VelX; VelY; 0]);  
acc = ([AccX;AccY;0]);
Rad = [l_F, l_F, -l_R, -l_R; -track_width_front/2, track_width_front/2, -track_width_rear/2, track_width_rear/2; 0, 0, 0, 0];  %Abstand cog zu rad mitte


% v_r = omega*r - v_x
% wheelAngleLeft/Right: positiv bei Rechtskurve
% gierrate positiv bei rechtskurve

% define velocity vector for CoG
% vel(1) = x(1);
% vel(2) = x(2) - x(14)*v2o_x; % checken ob evtl Vorzeichen vertauscht werden muss
% vel(3) = 0;%TODO:wenn gefilterte, plausible Werte von Sensorfusion, dann hier dazunehmen

% define acceleration vector for CoG
% acc(1) = x(5);
% acc(2) = x(6);
% acc(3) = 0;%TODO:wenn gefilterte, plausible Werte von Sensorfusion, dann hier dazunehmen

% define yaw rate and yaw acceleration of CoG
% yawRate = x(15);
% yawAcc = x(16); 

%% Rösselsprung-Matrizen für Rotation
% omegaTilde = [0,-YawRate,PitchRate;  
%                 YawRate,0,-RollRate;
%                     -PitchRate,RollRate,0];
% omegaDotTilde = [0,-YawAcc,PitchAcc;
%                    YawAcc,0,-RollAcc;
%                     -PitchAcc,RollAcc,0];
%        
omegaTilde = [0,-YawRate,0;...  % hier eigentlich noch Pitch und roll rate
                YawRate,0,0;...
                    0,0,0];
omegaDotTilde = [0,-YawAcc,0;...
                   YawAcc,0,0;...
                    0,0,0];                

% velocity of tires 
velTire_FL = vel + omegaTilde * Rad(:,1);
velTire_FR = vel + omegaTilde * Rad(:,2);
velTire_RL = vel + omegaTilde * Rad(:,3);
velTire_RR = vel + omegaTilde * Rad(:,4);

velTire = [velTire_FL; velTire_FR; velTire_RL; velTire_RR];
% acceleration of tires %TODO: Passende Formel aus
% Maschinendynamik raussuchen und verifizieren
accTire_FL = acc + omegaDotTilde * Rad(:,1) + omegaTilde * (omegaTilde * Rad(:,1)); 
accTire_FR = acc + omegaDotTilde * Rad(:,2) + omegaTilde * (omegaTilde * Rad(:,2));
accTire_RL = acc + omegaDotTilde * Rad(:,3) + omegaTilde * (omegaTilde * Rad(:,3));
accTire_RR = acc + omegaDotTilde * Rad(:,4) + omegaTilde * (omegaTilde * Rad(:,4));

accTire= [accTire_FL; accTire_FR; accTire_RL; accTire_RR];

%% Rotational matrices for Transformation from car coordinate system 
% into wheel coordinate systems
% rotMatrix_Front = [cos(delta),sin(delta),0; ... % hier eigentlich auch noch roll und pitch angle
%               -sin(delta),cos(delta),0;...
%               0,0,1];
          
rotMatrix_FL = [cos(WheelAngle_FL),sin(WheelAngle_FL),0; ... % hier eigentlich auch noch roll und pitch angle
              -sin(WheelAngle_FL),cos(WheelAngle_FL),0;...
              0,0,1];
          
rotMatrix_FR = [cos(WheelAngle_FR),sin(WheelAngle_FR),0; ... % hier eigentlich auch noch roll und pitch angle
              -sin(WheelAngle_FR),cos(WheelAngle_FR),0;...
              0,0,1];
rotMatrix_Rear = [1,0,0; 0,1,0; 0,0,1];
          
          
%% Transformationsmatrixen von Vehicle cog zu den einzelnen Rädern mit Roll und Pitchangle
% inverse von (11.9 und 11.10) für vorne und hinten
% rotMatrix_Front=[cos(delta)*cos(PitchAngle),-sin(delta)*cos(PitchAngle),-sin(PitchAngle);  % hier eigentlich auch noch roll und pitch angle
%               sin(RollAngle)*sin(PitchAngle)*cos(delta)-sin(delta)*cos(RollAngle),...
%               -sin(RollAngle)*sin(PitchAngle)*sin(WheelAngle(1)+cos(WheelAngle(1))*cos(RollAngle),...
%               sin(RollAngle)*cos(PitchAngle));
%               cos(RollAngle)*sin(PitchAngle)*cos(delta)-sin(RollAngle)*sin(delta),...
%                   -cos(RollAngle)*sin(PitchAngle)*sin(delta)-sin(RollAngle)*cos(delta),cos(RollAngle)*cos(PitchAngle)];
% 
% rotMatrix_Rear=([cos(PitchAngle),0, -sin(PitchAngle); 
%               sin(RollAngle)*sin(PitchAngle),cos(RollAngle),sin(RollAngle)*cos(PitchAngle);
%               cos(RollAngle)*sin(PitchAngle),-sin(RollAngle), cos(RollAngle)*cos(PitchAngle)]);
%%


% velocity of tires in tire coordinats (dieses Superpositionsprinzip ändert sich bei beta
% ungleich 0)
% wenn andere transformationsmatrix * durhch \ ersetzen
vel_help_FL = rotMatrix_FL * velTire_FL;
velX_FL = vel_help_FL(1);
velY_FL = vel_help_FL(2);
vel_help_FR = rotMatrix_FR* velTire_FR;
velX_FR = vel_help_FR(1);
velY_FR = vel_help_FR(2);
vel_help_RL = rotMatrix_Rear*velTire_RL;
velX_RL = vel_help_RL(1);
velY_RL = vel_help_RL(2);
vel_help_RR = rotMatrix_Rear*velTire_RR;
velX_RR = vel_help_RR(1);
velY_RR = vel_help_RR(2);

velX= single([velX_FL, velX_FR, velX_RL, velX_RR]);
velY= single([velY_FL, velY_FR, velY_RL, velY_RR]);

% acceleration of tires in tire coordinates
acc_FL = rotMatrix_FL * accTire_FL;
accX_FL = acc_FL(1);
acc_FR = rotMatrix_FR* accTire_FR;
accX_FR = acc_FR(1);
acc_RL = rotMatrix_Rear* accTire_RL;
accX_RL = acc_RL(1);
acc_RR = rotMatrix_Rear*accTire_RR;
accX_RR = acc_RR(1);
accX=[accX_FL, accX_FR, accX_RL, accX_RR];

% relative velocities of wheels
velRelX_FL = WheelVelocity_FL - velX_FL;  %hier später die Zustände aus dem kalman filter für wheelspeeds
velRelX_FR = WheelVelocity_FR - velX_FR;
velRelX_RL = WheelVelocity_RL  - velX_RL;
velRelX_RR = WheelVelocity_RR  - velX_RR;

velRelX= [velRelX_FL; velRelX_FR; velRelX_RL; velRelX_RR];

% e=100;
% TireSlipLong_BMW = [(velRelX_FL/(0.5*(sqrt(WheelVelocity_FL+e)+ sqrt(velX_FL+e)+ sqrt(sqrt((WheelVelocity_FL)+e) - sqrt(velX_FL+e)+ e)))); ...
%         (velRelX_FR/(0.5*(sqrt(WheelVelocity_FR+e)+ sqrt(velX_FR+e)+ sqrt(sqrt((WheelVelocity_FR)+e) - sqrt(velX_FR+e)+ e))));...
%         (velRelX_RL/(0.5*(sqrt(WheelVelocity_RL+e)+ sqrt(velX_RL+e)+ sqrt(sqrt((WheelVelocity_RL)+e) - sqrt(velX_RL+e)+ e))));...
%         (velRelX_RR/(0.5*(sqrt(WheelVelocity_RR+e)+ sqrt(velX_RR+e)+ sqrt(sqrt((WheelVelocity_RR)+e) - sqrt(velX_RR+e)+ e))))]; 
if(velX*ones(4,1) < 0.4) %TODO: Nachschauen, ob die Schwelle Probleme bereitet, oder ob diese höher oder tiefer gesetzt werden muss
    TireSlipLong = single([0, 0, 0, 0].');
else    		
TireSlipLong = [(velRelX_FL/max(abs(velX_FL), abs(WheelVelocity_FL))); (velRelX_FR/max(abs(velX_FR), abs(WheelVelocity_FR)));...
        (velRelX_RL/max(abs(velX_RL), abs(WheelVelocity_RL)));(velRelX_RR/max(abs(velX_RR), abs(WheelVelocity_RR)))];
end   

% zeta_test=(VelX-13)/(15-13); 
% zeta=(VelX-13)/(15-13); 
% if zeta_test > 1
%    zeta=single(1);
% elseif zeta_test < 0
%    zeta = single(0);
% end
% 
% 
% if(velX*ones(4,1) < 0.4) %TODO: Nachschauen, ob die Schwelle Probleme bereitet, oder ob diese höher oder tiefer gesetzt werden muss
%     TireSlipLong_TC = single([0, 0, 0, 0].');
% else
%     TireSlipLong_TC = [(velRelX_FL/(0.5*(sqrt(WheelVelocity_FL+e)+ sqrt(velX_FL+e)+ sqrt(sqrt((WheelVelocity_FL)+e) - sqrt(velX_FL+e)+ e))))*(1-zeta)+zeta*(velRelX_FL/max(abs(velX_FL), abs(WheelVelocity_FL))); ...
%         (velRelX_FR/(0.5*(sqrt(WheelVelocity_FR+e)+ sqrt(velX_FR+e)+ sqrt(sqrt((WheelVelocity_FR)+e) - sqrt(velX_FR+e)+ e))))*(1-zeta)+zeta*(velRelX_FR/max(abs(velX_FR), abs(WheelVelocity_FR)));...
%         (velRelX_RL/(0.5*(sqrt(WheelVelocity_RL+e)+ sqrt(velX_RL+e)+ sqrt(sqrt((WheelVelocity_RL)+e) - sqrt(velX_RL+e)+ e))))*(1-zeta)+zeta*(velRelX_RL/max(abs(velX_RL), abs(WheelVelocity_RL)));...
%         (velRelX_RR/(0.5*(sqrt(WheelVelocity_RR+e)+ sqrt(velX_RR+e)+ sqrt(sqrt((WheelVelocity_RR)+e) - sqrt(velX_RR+e)+ e))))*(1-zeta)+zeta*(velRelX_RR/max(abs(velX_RR), abs(WheelVelocity_RR)))];
% 
% %     TireSlipLong = [(velRelX_FL/max(abs(velX_FL), abs(WheelVelocity_FL))); (velRelX_FR/max(abs(velX_FR), abs(WheelVelocity_FR)));...
% %         (velRelX_RL/max(abs(velX_RL), abs(WheelVelocity_RL)));(velRelX_RR/max(abs(velX_RR), abs(WheelVelocity_RR)))];
% end
% if switch_TireSlip_pGL==0
%     TireSlipLong_TC=TireSlipLong;
% end

if(velX*ones(4,1) < 0.4)
    TireSlipAngle = single([0, 0, 0, 0].');
else
     TireSlipAngle = [-atan(velY_FL)/(abs(velX_FL)); ...
        -atan(velY_FR)/(abs(velX_FR));... % hier müssen dann die Zustände von kalman mit mal r übertragen werden
        -atan(velY_RL)/(abs(velX_RL));...
       -atan(velY_RR)/(abs(velX_RR))];
%         TireSlipAngle = [-atan(velY_FL)/(abs(WheelVelocity_FL)); ...
%         -atan(velY_FR)/(abs(WheelVelocity_FR);... % hier müssen dann die Zustände von kalman mit mal r übertragen werden
%         -atan(velY_RL)/(abs(WheelVelocity_RL);...
%        -atan(velY_RR)/(abs(WheelVelocity_RR)];
   
end

% for n=1:1:4
%     if TireSlipLong_TC(n) > 1
%         TireSlipLong_TC(n) = 1;
%     elseif TireSlipLong_TC(n) < -1
%         TireSlipLong_TC(n) = -1;
%     end
% end

for n=1:1:4
    if TireSlipLong(n) > 1
        TireSlipLong(n) = 1;
    elseif TireSlipLong(n) < -1
        TireSlipLong(n) = -1;
    end
end
%mit v=omega*r und alpha=omega/t=omega*r/(t*r)=a/r
WheelSpeedNoSlip = velX.'/(tire_r_dyn);
WheelAccNoSlip = accX.'/(tire_r_dyn);

end
